simulink model "DiodeRectifier_Rload"  (R2018b)
settings: Solver=VariableStepAuto  StartTime=0.0  StopTime=0.10  RelTol=1e-3
libraries: powerlib x18
settings Model: Creator=A.hey  LastModifiedBy=A.hey

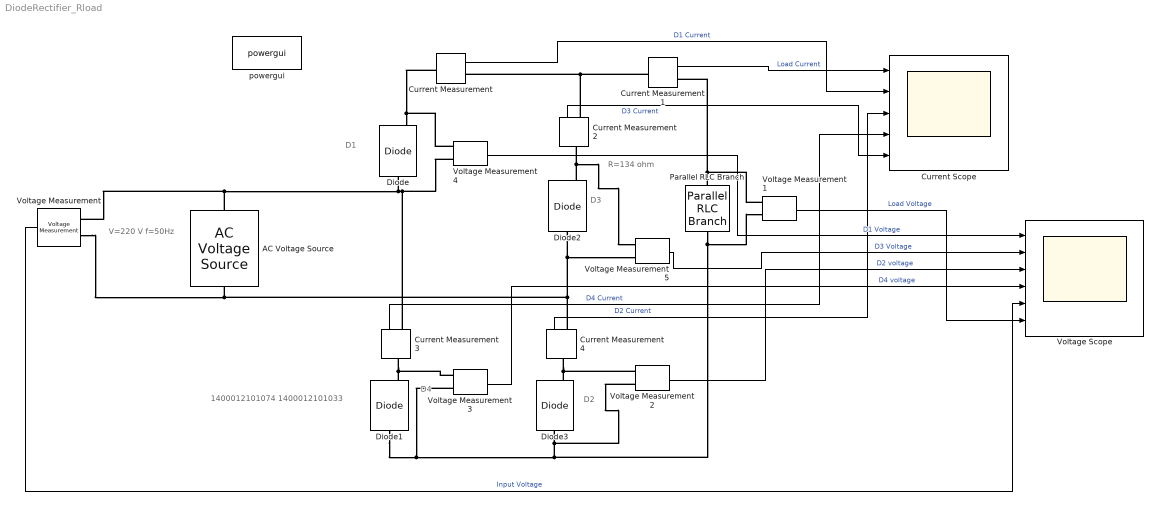
== system DiodeRectifier_Rload ==
  note: V=220 V
      | f=50Hz
  note: R=134 ohm
  note: D1
  note: D2
  note: D4
  note: D3
  note: 1400012101074
      | 1400012101033
  AC Voltage Source : powerlib/Electrical Sources/AC Voltage Source  Amplitude=220  Phase=0  Frequency=50  SampleTime=0  Measurements=None  BusType=swing  Pref=10e3  Qref=0  Qmin=-inf  Qmax=+inf
  Current Measurement{,1..4} (5 alike) : powerlib/Measurements/Current Measurement  PhasorSimulation=off  OutputType=Complex  PSBequivalent=0
  Current Scope : Scope  NumInputPorts=5
  Diode{,1..3} (4 alike) : powerlib/Power Electronics/Diode  Ron=0.001  Lon=0  Vf=0.8  IC=0  UseSnubber=0  Rs=500  Cs=250e-9  Measurements=on
  Parallel RLC Branch : powerlib/Elements/Parallel RLC Branch  LConnTagsString=a  RConnTagsString=__new0  BranchType=R  Resistance=134  Inductance=1e-3  SetiL0=off  InitialCurrent=0  Capacitance=1e-6  Setx0=off  InitialVoltage=0  Measurements=None
  Voltage Measurement{,1..5} (6 alike) : powerlib/Measurements/Voltage Measurement  PhasorSimulation=off  OutputType=Complex  PSBequivalent=0
  "Voltage Scope " : Scope  NumInputPorts=6
  powergui : powerlib/powergui  Priority=1  SimulationMode=Continuous  SampleTime=50e-6  frequency=60  Iterations=50  frequencyindice=50  Pbase=100e6  ErrMax=1e-4  UnitsV=kV  UnitsW=MW  buscounter=0  FunctionMessages=off  echomessages=off  EnableUseOfTLC=off  CurrentSourceSwitches=off  DisableSnubberDevices=off  DisableRonSwitches=off  DisableVfSwitches=off  DisplayEquations=off  SolverType=Tustin/Backward Euler (TBE)  Interpol=off  ExternalGateDelay=off  methode=off  Ts=100  x0status=blocks  SPID=on  SwTol=0  HookPort=off  RestoreLinks=warning  ResistiveCurrentMeasurement=off  Frange=[0:2:500]  Ylog=off  Xlog=on  ShowGrid=off  save=off  variable=ZData  structure=0  ZoomFFT=off  StartTime=0.0  cycles=1  DisplayStyle=1  fundamental=60  FreqAxis=off  MaxFrequency=1000  frequencyindicesteady=1  RmsSteady=1  display=off
  wires:
  Current Measurement1/1 -> Current Scope/1  "Load Current"
  Current Measurement/1 -> Current Scope/2  "D1 Current"
  Current Measurement4/1 -> Current Scope/3  "D2 Current"
  Current Measurement3/1 -> Current Scope/4  "D4 Current"
  Current Measurement2/1 -> Current Scope/5  "D3 Current"
  Voltage Measurement5/1 -> "Voltage Scope "/2  "D3 Voltage"
  Voltage Measurement4/1 -> "Voltage Scope "/1  "D1 Voltage"
  Voltage Measurement2/1 -> "Voltage Scope "/3  "D2 voltage"
  Voltage Measurement3/1 -> "Voltage Scope "/4  "D4 voltage"
  Voltage Measurement1/1 -> "Voltage Scope "/6  "Load Voltage"
  Voltage Measurement/1 -> "Voltage Scope "/5  "Input Voltage"
  connections:
  AC Voltage Source/RConn1 -- Voltage Measurement/LConn1 -- Voltage Measurement4/LConn1 -- Current Measurement3/RConn1 -- Diode/LConn1
  Parallel RLC Branch/LConn1 -- Current Measurement1/RConn1 -- Voltage Measurement1/LConn1
  Diode3/RConn1 -- Voltage Measurement2/LConn2 -- Current Measurement4/LConn1
  Diode1/LConn1 -- Voltage Measurement3/LConn1 -- Voltage Measurement1/LConn2 -- Parallel RLC Branch/RConn1 -- Voltage Measurement2/LConn1 -- Diode3/LConn1
  Current Measurement/LConn1 -- Voltage Measurement4/LConn2 -- Diode/RConn1
  Diode2/RConn1 -- Voltage Measurement5/LConn2 -- Current Measurement2/LConn1
  Current Measurement1/LConn1 -- Current Measurement/RConn1 -- Current Measurement2/RConn1
  Diode1/RConn1 -- Voltage Measurement3/LConn2 -- Current Measurement3/LConn1
  Current Measurement4/RConn1 -- Voltage Measurement5/LConn1 -- Diode2/LConn1 -- Voltage Measurement/LConn2 -- AC Voltage Source/LConn1
